simulink model "sampleModel1646"  (R2023a)
settings: Solver=VariableStepAuto  StartTime=0.0  StopTime=10.0  RelTol=1e-3
libraries: hdlsllib x7, simulink x1
settings Model: Creator=user1  LastModifiedBy=user1

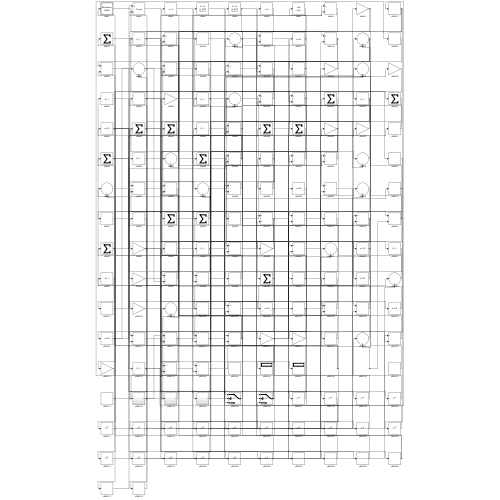
[thumbnail: Simulink's stored preview of the top-level diagram]
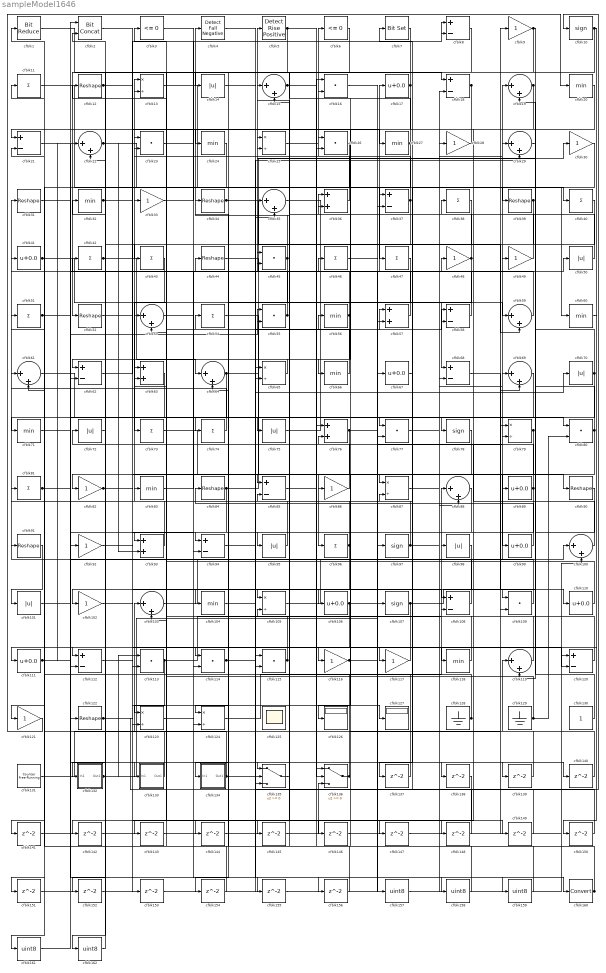
== system sampleModel1646 ==
  cfblk1 : hdlsllib/Logic and Bit Operations/Bit Reduce  mode=AND
  cfblk{10,78,97,107} (4 alike) : Signum
  cfblk{15,19,22,29,35,53,59,61,64,69,88,100,103,119} (14 alike) : Sum  Inputs=|++
  cfblk{14,50,70,72,75,95,98,101} (8 alike) : Abs  SaturateOnIntegerOverflow=off
  cfblk{9,28,30,33,48..49,82,86,92,102,116..117,121} (13 alike) : Gain
  cfblk{20,24,27,32,56,60,66,71,83,104,118} (11 alike) : MinMax
  cfblk{13,25,65,79,87,105,123..124} (8 alike) : Product  Inputs=*/  RndMeth=Zero  SaturateOnIntegerOverflow=on
  cfblk{17,41,67,89,99,106,110..111} (8 alike) : Bias  Bias=0.0  SaturateOnIntegerOverflow=off
  cfblk{8,18,21,37,58,62,68,85,94,108,112,120} (12 alike) : Sum  Inputs=+-
  cfblk{16,23,26,45,55,77,80,109,113..115} (11 alike) : DotProduct  OutDataTypeStr=Inherit: Inherit via internal rule
  cfblk{11,38,40,42..43,46..47,51,54,73..74,81,96} (13 alike) : Sum  Inputs=+
  cfblk{12,31,34,39,44,52,84,90..91,122} (10 alike) : Reshape
  cfblk125 : Scope
      settings: Floating=on
  cfblk126 : Display
  cfblk127 : Display
  cfblk128 : Ground
  cfblk129 : Ground
  cfblk130 : Constant  SampleTime=-1
  cfblk131 : hdlsllib/Sources/Counter Free-Running  NumBits=16  tsamp=-1
  cfblk132 : Subsystem
      settings: LibrarySourceBlock=|
      | hdlsllib/Ports &
      | Subsystems/Subsystem
  cfblk133 : Subsystem
      settings: LibrarySourceBlock=|
      | hdlsllib/Ports &
      | Subsystems/Subsystem
  cfblk134 : Subsystem
      settings: LibrarySourceBlock=|
      | hdlsllib/Ports &
      | Subsystems/Subsystem
  cfblk135 : Switch  SaturateOnIntegerOverflow=off  InputSameDT=off
  cfblk136 : Switch  SaturateOnIntegerOverflow=off  InputSameDT=off
  cfblk{137..156} (20 alike) : Delay  SampleTime=1
  cfblk{157..159,161..162} (5 alike) : DataTypeConversion  OutDataTypeStr=uint8  SaturateOnIntegerOverflow=off  RndMeth=Floor
  cfblk160 : DataTypeConversion  SaturateOnIntegerOverflow=off  RndMeth=Floor
  cfblk2 : hdlsllib/Logic and Bit Operations/Bit Concat  numInputs=2
  cfblk3 : hdlsllib/Logic and Bit Operations/Compare To Zero  relop=<=  OutDataTypeStr=boolean
  cfblk{36,57,63,76,93} (5 alike) : Sum
  cfblk4 : hdlsllib/Logic and Bit Operations/Detect Fall Negative  vinit=0  OutDataTypeStr=boolean
  cfblk5 : hdlsllib/Logic and Bit Operations/Detect Rise Positive  vinit=0  OutDataTypeStr=boolean
  cfblk6 : hdlsllib/Logic and Bit Operations/Compare To Zero  relop=<=  OutDataTypeStr=boolean
  cfblk7 : simulink/Logic and Bit Operations/Bit Set  iBit=0
      settings: LibrarySourceBlock=|
      | hdlsllib/Logic and Bit
      | Operations/Bit Set
  wires:
  cfblk99/1 -> cfblk84/1
  cfblk93/1 -> cfblk13/1
  cfblk27/1 -> cfblk52/1, cfblk124/2
  cfblk115/1 -> cfblk31/1, cfblk81/1
  cfblk58/1 -> cfblk7/1
  cfblk96/1 -> cfblk33/1, cfblk115/2
  cfblk45/1 -> cfblk4/1, cfblk65/2
  cfblk90/1 -> cfblk105/1
  cfblk43/1 -> cfblk73/1
  cfblk41/1 -> cfblk68/1, cfblk135/1, cfblk94/2, cfblk75/1
  cfblk36/1 -> cfblk5/1
  cfblk10/1 -> cfblk116/1, cfblk132/1(In1), cfblk154/1
  cfblk134/1(Out1) -> cfblk103/1, cfblk70/1
  cfblk51/1 -> cfblk122/1, cfblk156/1
  cfblk57/1 -> cfblk17/1
  cfblk122/1 -> cfblk10/1, cfblk155/1
  cfblk26/1 -> cfblk121/1
  cfblk75/1 -> cfblk78/1
  cfblk2/1 -> cfblk160/1
  cfblk84/1 -> cfblk58/1, cfblk113/2
  cfblk124/1 -> cfblk88/1
  cfblk76/1 -> cfblk96/1, cfblk120/2, cfblk152/1
  cfblk128/1 -> cfblk34/1, cfblk45/2
  cfblk79/1 -> cfblk76/2, cfblk123/2
  cfblk37/1 -> cfblk6/1, cfblk85/1
  cfblk100/1 -> cfblk72/1
  cfblk69/1 -> cfblk77/1
  cfblk132/1(Out1) -> cfblk67/1, cfblk113/1
  cfblk21/1 -> cfblk92/1
  cfblk42/1 -> cfblk64/1, cfblk87/1
  cfblk121/1 -> cfblk20/1
  cfblk67/1 -> cfblk117/1
  cfblk17/1 -> cfblk21/1, cfblk14/1
  cfblk95/1 -> cfblk83/1
  cfblk72/1 -> cfblk102/1
  cfblk130/1 -> cfblk38/1
  cfblk61/1 -> cfblk97/1
  cfblk101/1 -> cfblk100/1
  cfblk129/1 -> cfblk13/2, cfblk80/2
  cfblk108/1 -> cfblk98/1
  cfblk107/1 -> cfblk109/1, cfblk112/1
  cfblk116/1 -> cfblk58/2, cfblk79/2
  cfblk35/1 -> cfblk107/1
  cfblk102/1 -> cfblk118/1
  cfblk47/1 -> cfblk94/1
  cfblk119/1 -> cfblk91/1
  cfblk6/1 -> cfblk43/1
  cfblk105/1 -> cfblk19/1
  cfblk87/1 -> cfblk69/1
  cfblk64/1 -> cfblk30/1, cfblk112/2
  cfblk55/1 -> cfblk25/1, cfblk22/2
  cfblk110/1 -> cfblk63/1
  cfblk15/1 -> cfblk40/1, cfblk145/1
  cfblk77/1 -> cfblk50/1
  cfblk49/1 -> cfblk15/1
  cfblk66/1 -> cfblk41/1
  cfblk88/1 -> cfblk95/1
  cfblk131/1 -> cfblk109/2
  cfblk54/1 -> cfblk86/1
  cfblk136/1 -> cfblk32/1, cfblk61/1
  cfblk53/1 -> cfblk59/1
  cfblk50/1 -> cfblk36/1
  cfblk104/1 -> cfblk56/1
  cfblk18/1 -> cfblk66/1, cfblk37/2
  cfblk11/1 -> cfblk39/1
  cfblk5/1 -> cfblk136/2, cfblk53/2
  cfblk73/1 -> cfblk99/1
  cfblk85/1 -> cfblk57/1
  cfblk25/1 -> cfblk26/1
  cfblk9/1 -> cfblk89/1, cfblk15/2
  cfblk71/1 -> cfblk45/1
  cfblk12/1 -> cfblk27/1, cfblk90/1
  cfblk117/1 -> cfblk111/1
  cfblk22/1 -> cfblk60/1, cfblk93/2
  cfblk3/1 -> cfblk108/1
  cfblk80/1 -> cfblk25/2, cfblk71/1, cfblk126/1
  cfblk62/1 -> cfblk8/1
  cfblk7/1 -> cfblk26/2
  cfblk38/1 -> cfblk57/2
  cfblk109/1 -> cfblk42/1
  cfblk13/1 -> cfblk47/1
  cfblk91/1 -> cfblk101/1
  cfblk40/1 -> cfblk82/1
  cfblk97/1 -> cfblk29/1, cfblk51/1
  cfblk70/1 -> cfblk19/2, cfblk114/2
  cfblk14/1 -> cfblk80/1
  cfblk29/1 -> cfblk119/2
  cfblk19/1 -> cfblk53/1, cfblk93/1, cfblk148/1
  cfblk20/1 -> cfblk74/1
  cfblk103/1 -> cfblk9/1
  cfblk33/1 -> cfblk8/2
  cfblk106/1 -> cfblk48/1, cfblk135/2
  cfblk28/1 -> cfblk24/1
  cfblk59/1 -> cfblk3/1
  cfblk133/1(Out1) -> cfblk11/1
  cfblk1/1 -> cfblk18/1
  cfblk83/1 -> cfblk49/1
  cfblk48/1 -> cfblk23/1, cfblk104/1, cfblk114/1
  cfblk89/1 -> cfblk124/1, cfblk55/2
  cfblk31/1 -> cfblk133/1(In1)
  cfblk39/1 -> cfblk134/1(In1), cfblk144/1
  cfblk32/1 -> cfblk127/1, cfblk139/1
  cfblk135/1 -> cfblk105/2
  cfblk34/1 -> cfblk59/2, cfblk64/2
  cfblk114/1 -> cfblk65/1, cfblk44/1
  cfblk78/1 -> cfblk103/2
  cfblk120/1 -> cfblk12/1
  cfblk113/1 -> cfblk123/1, cfblk108/2
  cfblk86/1 -> cfblk35/1
  cfblk65/1 -> cfblk62/1
  cfblk94/1 -> cfblk29/2
  cfblk81/1 -> cfblk55/1, cfblk151/1
  cfblk111/1 -> cfblk62/2, cfblk22/1
  cfblk68/1 -> cfblk110/1
  cfblk56/1 -> cfblk23/2, cfblk135/3
  cfblk82/1 -> cfblk106/1, cfblk146/1
  cfblk118/1 -> cfblk37/1
  cfblk74/1 -> cfblk21/2
  cfblk44/1 -> cfblk46/1
  cfblk30/1 -> cfblk137/1
  cfblk137/1 -> cfblk1/1
  cfblk112/1 -> cfblk138/1
  cfblk139/1 -> cfblk36/2
  cfblk92/1 -> cfblk140/1
  cfblk140/1 -> cfblk119/1
  cfblk24/1 -> cfblk141/1
  cfblk141/1 -> cfblk69/2
  cfblk98/1 -> cfblk142/1
  cfblk142/1 -> cfblk68/2
  cfblk8/1 -> cfblk143/1
  cfblk143/1 -> cfblk100/2
  cfblk144/1 -> cfblk136/3
  cfblk145/1 -> cfblk136/1
  cfblk146/1 -> cfblk79/1
  cfblk23/1 -> cfblk147/1
  cfblk147/1 -> cfblk88/2
  cfblk148/1 -> cfblk87/2
  cfblk46/1 -> cfblk149/1
  cfblk149/1 -> cfblk76/1
  cfblk60/1 -> cfblk150/1
  cfblk150/1 -> cfblk115/1
  cfblk151/1 -> cfblk35/2
  cfblk152/1 -> cfblk77/2
  cfblk52/1 -> cfblk153/1
  cfblk153/1 -> cfblk120/1
  cfblk154/1 -> cfblk61/2
  cfblk155/1 -> cfblk18/2
  cfblk156/1 -> cfblk63/2
  cfblk16/1 -> cfblk157/1
  cfblk157/1 -> cfblk28/1
  cfblk123/1 -> cfblk158/1
  cfblk158/1 -> cfblk16/1
  cfblk4/1 -> cfblk159/1
  cfblk159/1 -> cfblk16/2
  cfblk160/1 -> cfblk85/2, cfblk54/1
  cfblk63/1 -> cfblk161/1
  cfblk161/1 -> cfblk2/1
  cfblk138/1 -> cfblk162/1
  cfblk162/1 -> cfblk2/2

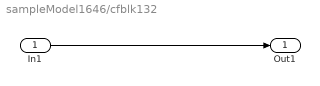
== system sampleModel1646/cfblk132 ==
  In1 : Inport
  Out1 : Outport
  wires:
  In1/1 -> Out1/1

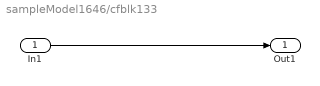
== system sampleModel1646/cfblk133 ==
  In1 : Inport
  Out1 : Outport
  wires:
  In1/1 -> Out1/1

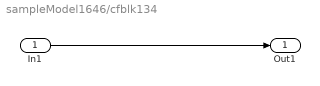
== system sampleModel1646/cfblk134 ==
  In1 : Inport
  Out1 : Outport
  wires:
  In1/1 -> Out1/1
